simulink model "project_2_CentitoFaren"  (R2023a)
settings: Solver=VariableStepAuto  StartTime=0.0  StopTime=10.0  RelTol=1e-3
values from neighbouring files (symbols this model uses):
  x = input('enter T in C ')    [project_2_CentitoFaren_script.m]
settings Model: Creator=FC  LastModifiedBy=FC

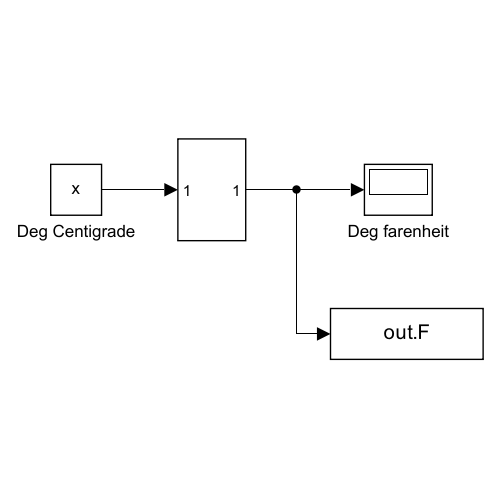
[thumbnail: Simulink's stored preview of the top-level diagram]
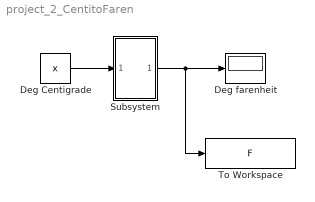
== system project_2_CentitoFaren ==
  Deg Centigrade : Constant  Value=x
  Deg farenheit : Display
  Subsystem : Subsystem
  To Workspace : ToWorkspace  VariableName=F  SampleTime=-1
      settings: Save2DSignal=2-D array (concatenate along first dimension)
  wires:
  Deg Centigrade/1 -> Subsystem/1(In1)
  Subsystem/1(Out1) -> To Workspace/1, Deg farenheit/1

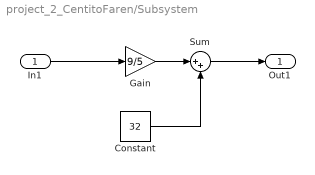
== system project_2_CentitoFaren/Subsystem ==
  In1 : Inport
  Constant : Constant  Value=32
  Gain : Gain  Gain=9/5
  Sum : Sum  Inputs=|++
  Out1 : Outport
  wires:
  Gain/1 -> Sum/1
  Constant/1 -> Sum/2
  In1/1 -> Gain/1
  Sum/1 -> Out1/1
